simulink model "Voltage_Current_Dividers"  (R2019b)
settings: Solver=VariableStepAuto  StartTime=0.0  StopTime=10.0  MaxStep=1e-4  RelTol=1e-4
libraries: powerlib x15
settings Model: Creator=eprie  LastModifiedBy=eprie

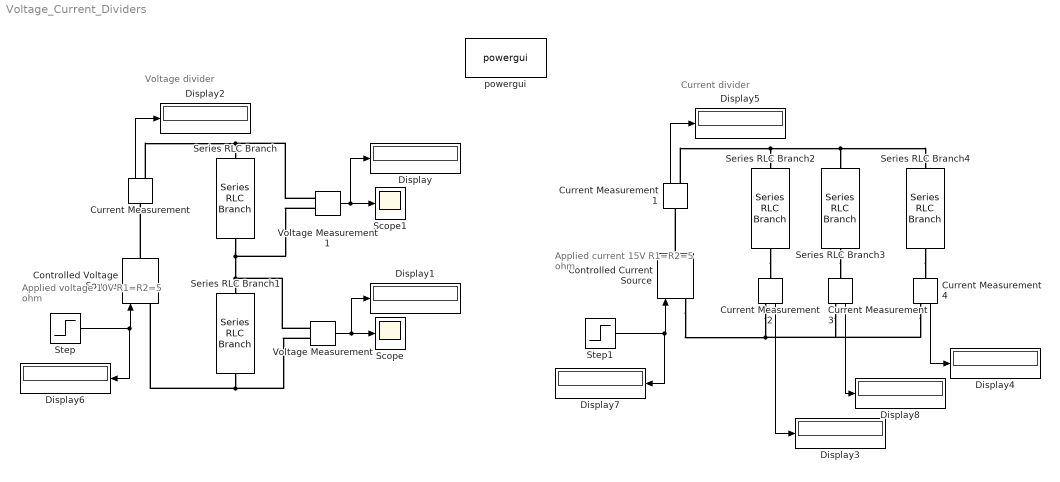
== system Voltage_Current_Dividers ==
  note: Voltage divider
  note: Applied voltage 10V
      | R1=R2=5 ohm
  note: Applied current 15V
      | R1=R2=5 ohm
  note: Current divider
  Controlled Current Source : powerlib/Electrical Sources/Controlled Current Source  Initialize=off  Source_Type=DC  Amplitude=15  Phase=0  Frequency=0  Measurements=None
      settings: SourceProductName=Simscape Electrical
  Controlled Voltage Source : powerlib/Electrical Sources/Controlled Voltage Source  Initialize=on  Source_Type=AC  Amplitude=0  Phase=0  Frequency=0  Measurements=None
      settings: SourceProductName=Simscape Electrical
  Current Measurement{,1..4} (5 alike) : powerlib/Measurements/Current Measurement  PhasorSimulation=off  OutputType=Complex  PSBequivalent=0
      settings: SourceProductName=Simscape Electrical
  Display{,1..8} (9 alike) : Display
  Scope : Scope
  Scope1 : Scope
  Series RLC Branch{,1..4} (5 alike) : powerlib/Elements/Series RLC Branch  LConnTagsString=__new0  RConnTagsString=__new0  BranchType=R  Resistance=5  Inductance=1e-3  SetiL0=off  InitialCurrent=0  Capacitance=1e-6  Setx0=off  InitialVoltage=0  Measurements=None
      settings: SourceProductName=Simscape Electrical
  Step : Step  Time=0  After=10  SampleTime=0
  Step1 : Step  Time=0  After=15  SampleTime=0
  Voltage Measurement : powerlib/Measurements/Voltage Measurement  PhasorSimulation=off  OutputType=Complex  PSBequivalent=0
      settings: SourceProductName=Simscape Electrical
  Voltage Measurement1 : powerlib/Measurements/Voltage Measurement  PhasorSimulation=off  OutputType=Complex  PSBequivalent=0
      settings: SourceProductName=Simscape Electrical
  powergui : powerlib/powergui  Priority=1  SimulationMode=Continuous  SampleTime=50e-6  frequency=60  Iterations=50  frequencyindice=0  Pbase=100e6  ErrMax=1e-4  UnitsV=kV  UnitsW=MW  buscounter=0  FunctionMessages=off  echomessages=off  EnableUseOfTLC=off  CurrentSourceSwitches=off  DisableSnubberDevices=off  DisableRonSwitches=off  DisableVfSwitches=off  DisplayEquations=off  AutomaticDiscreteSolvers=off  SolverType=Tustin/Backward Euler (TBE)  Interpol=off  ExternalGateDelay=off  methode=off  Ts=100  x0status=blocks  SPID=on  SwTol=0  HookPort=off  NonlinearTolerance=1e-4  nMaxIteration=100  ContinueOnMaxIteration=off  RestoreLinks=warning  ResistiveCurrentMeasurement=off  Frange=[0:2:500]  Ylog=off  Xlog=on  ShowGrid=off  save=off  variable=ZData  structure=0  ZoomFFT=off  StartTime=0.0  cycles=1  DisplayStyle=1  fundamental=60  FreqAxis=off  MaxFrequency=1000  frequencyindicesteady=1  RmsSteady=1  display=off
      settings: SourceProductName=Simscape Electrical
  wires:
  Step/1 -> Display6/1, Controlled Voltage Source/1
  Voltage Measurement/1 -> Display1/1, Scope/1
  Voltage Measurement1/1 -> Display/1, Scope1/1
  Current Measurement/1 -> Display2/1
  Current Measurement1/1 -> Display5/1
  Step1/1 -> Controlled Current Source/1, Display7/1
  Current Measurement2/1 -> Display3/1
  Current Measurement4/1 -> Display4/1
  Current Measurement3/1 -> Display8/1
  connections:
  Voltage Measurement1/LConn1 -- Current Measurement/RConn1 -- Series RLC Branch/LConn1
  Voltage Measurement/LConn2 -- Controlled Voltage Source/LConn1 -- Series RLC Branch1/RConn1
  Series RLC Branch/RConn1 -- Voltage Measurement1/LConn2 -- Voltage Measurement/LConn1 -- Series RLC Branch1/LConn1
  Controlled Voltage Source/RConn1 -- Current Measurement/LConn1
  Current Measurement1/RConn1 -- Series RLC Branch3/LConn1 -- Series RLC Branch4/LConn1 -- Series RLC Branch2/LConn1
  Controlled Current Source/RConn1 -- Current Measurement1/LConn1
  Series RLC Branch2/RConn1 -- Current Measurement2/LConn1
  Current Measurement2/RConn1 -- Controlled Current Source/LConn1 -- Current Measurement3/RConn1 -- Current Measurement4/RConn1
  Series RLC Branch3/RConn1 -- Current Measurement3/LConn1
  Series RLC Branch4/RConn1 -- Current Measurement4/LConn1
